simulink model "sec2date_example"  (Simulink 8.2)
settings: Solver=ode45  StartTime=0.0  StopTime=24*3600+1  RelTol=1e-3
libraries: carnot x2
settings Model: Creator=drhf  LastModifiedBy=drhf

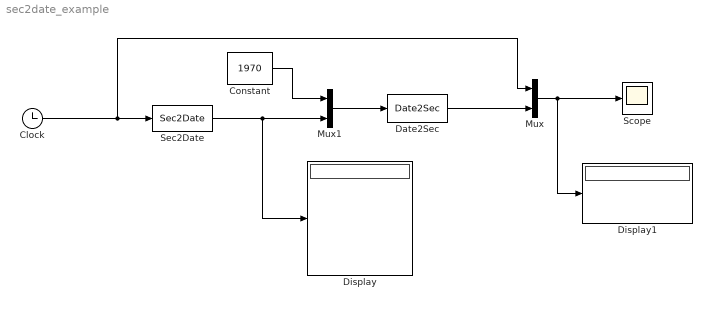
== system sec2date_example ==
  Clock : Clock
  Constant : Constant  Value=1970
  Date2Sec : carnot/Toolbox/Date2Sec
  Display : Display
  Display1 : Display
  Mux : Mux  Inputs=2
  Mux1 : Mux  Inputs=2
  Scope : Scope
  Sec2Date : carnot/Toolbox/Sec2Date
  wires:
  Sec2Date/1 -> Display/1, Mux1/2
  Clock/1 -> Sec2Date/1, Mux/1
  Date2Sec/1 -> Mux/2
  Mux/1 -> Display1/1, Scope/1
  Mux1/1 -> Date2Sec/1
  Constant/1 -> Mux1/1
